simulink model "kalman_filter_run"  (R2020b)
settings: Solver=FixedStepAuto  StartTime=0.0  StopTime=20  FixedStep=h  RelTol=1e-3  EnableMultiTasking=on
values from neighbouring files (symbols this model uses):
  R_kf = 1 * diag([1, 10, 1, 10])    [dc_motor_control.m]    (also in rotating_pendulum_3states.m = 10 * diag([1, 1, 10]); rotating_pendulum_4states.m = diag([7.5740e-06, 0.1526, 1.4489e-05, 0.2930]))
undefined symbols (not defined in the file or in its folder): Discrete, Time
libraries: ctrlSharedLib x1
settings Model: Creator=rbabuska  LastModifiedBy=danny
settings DataIOCC: LimitDataPoints=on  SaveFormat=Array  ReturnWorkspaceOutputs=off  SignalLoggingName=sigsOut
settings OptimizationCC: BooleanDataType=off  ExpressionDepthLimit=2147483647  InitFltsAndDblsToZero=on  LifeSpan=inf
settings DebuggingCC: SaveWithParameterizedLinksMsg=none  SignalResolutionControl=TryResolveAllWithWarning  MultiTaskDSMMsg=warning  MultiTaskCondExecSysMsg=none  AllowSymbolicDim=off  StateNameClashWarn=warning  SFUnexpectedBacktrackingDiag=warning  SFNoUnconditionalDefaultTransitionDiag=warning  SFExecutionAtInitializationDiag=none  ArithmeticOperatorsInVariantConditions=warning
settings HardwareCC: ProdBitPerPointer=32  ProdBitPerSizeT=32  ProdBitPerPtrDiffT=32  ProdLargestAtomicFloat=None  ProdIntDivRoundTo=Undefined  ProdEndianess=Unspecified  ProdWordSize=32  ProdHWDeviceType=32-bit Generic  TargetUnknown=on
settings ModelReferenceCC: PropagateSignalLabelsOutOfModel=off
settings SFSimCC: SimUseLocalCustomCode=off  CustomCodeUndefinedFunction=UseInterfaceOnly
settings RTWCC: RTWUseLocalCustomCode=off
settings CodeAppCC: StateflowObjectComments=on
settings GRTTargetCC: TargetFcnLib=ansi_tfl_tmw.mat  TargetLangStandard=C89/C90 (ANSI)  CombineOutputUpdateFcns=off  GRTInterface=on
settings ConfigComp: CovMetricSettings=dw  CovSaveCumulativeToWorkspaceVar=on  CovSaveSingleToWorkspaceVar=on  CovExternalEMLEnable=off

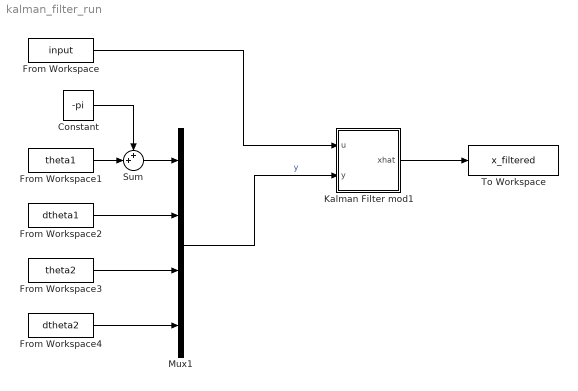
== system kalman_filter_run ==
  Constant : Constant  Value=-pi
  From Workspace : FromWorkspace  VariableName=input
  From Workspace1 : FromWorkspace  VariableName=theta1
  From Workspace2 : FromWorkspace  VariableName=dtheta1
  From Workspace3 : FromWorkspace  VariableName=theta2
  From Workspace4 : FromWorkspace  VariableName=dtheta2
  Kalman Filter mod1 : Subsystem
  Mux1 : Mux
  Sum : Sum  Inputs=++|
  To Workspace : ToWorkspace  VariableName=x_filtered  SaveFormat=Timeseries  SampleTime=-1
  wires:
  From Workspace/1 -> Kalman Filter mod1/1(u)
  Mux1/1 -> Kalman Filter mod1/2(y)  "y"
  From Workspace2/1 -> Mux1/2
  From Workspace4/1 -> Mux1/4
  From Workspace3/1 -> Mux1/3
  Kalman Filter mod1/1(xhat) -> To Workspace/1
  Sum/1 -> Mux1/1
  From Workspace1/1 -> Sum/2
  Constant/1 -> Sum/1

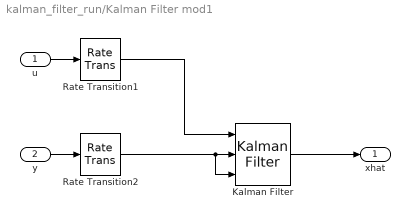
== system kalman_filter_run/Kalman Filter mod1 ==
  u : Inport
  y : Inport  Port=2
  Kalman Filter : ctrlSharedLib/Kalman Filter  TimeDomain=Discrete-Time  UseCurrentEstimator=on  ModelSource=LTI State-Space Variable  ModelSourceVariable=dt_sys_zoh  A=0.95  B=1  C=1  D=0  NumberOfStates=1  NumberOfInputs=1  NumberOfOutputs=1  InitialEstimateSource=Input port  X0=[0, 0, 0, 0]  P0=10  UseK=off  UseGH=off  NumberOfProcessNoiseInputs=1  G=1  TimeInvariantG=on  H=0  TimeInvariantH=on  Q=Q_kf  TimeInvariantQ=on  R=R_kf  TimeInvariantR=on  N=0  TimeInvariantN=on  AddInputPort=on  AddEnablePort=off  OutputEstimatedY=off  OutputP=off  Ts=-1
  Rate Transition1 : RateTransition
  Rate Transition2 : RateTransition
  xhat : Outport
  wires:
  y/1 -> Rate Transition2/1
  Kalman Filter/1 -> xhat/1
  u/1 -> Rate Transition1/1
  Rate Transition1/1 -> Kalman Filter/1
  Rate Transition2/1 -> Kalman Filter/2, Kalman Filter/3
